simulink model "manning_test_su_nonlinear"  (R2022b)
settings: Solver=VariableStepAuto  StartTime=0.0  StopTime=5*N  RelTol=1e-3
values from neighbouring files (symbols this model uses):
  yd_ds = ss(yd_ds)    [manning_test.m]
  yu_ds = ss(yu_ds)    [manning_test.m]
settings Model: Creator=chuan  LastModifiedBy=chuan

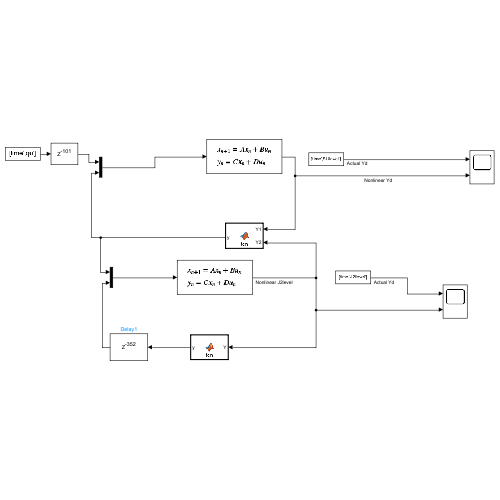
[thumbnail: Simulink's stored preview of the top-level diagram]
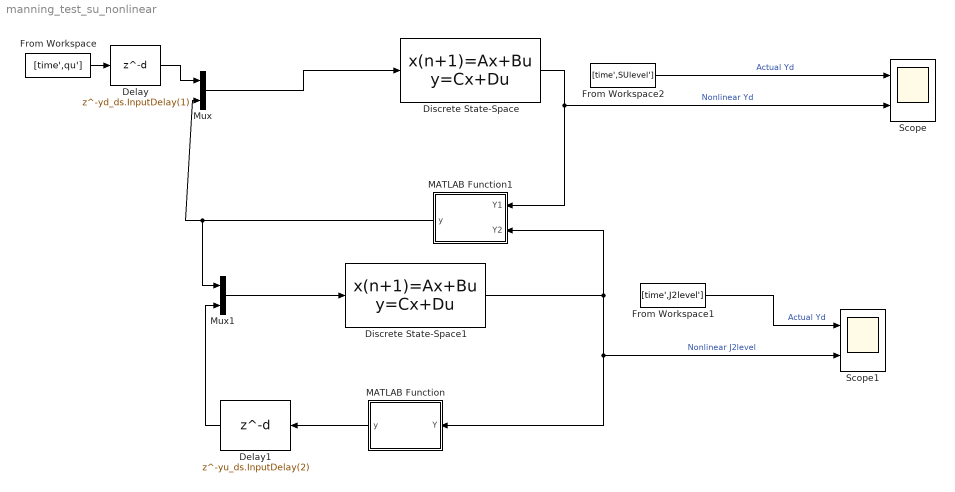
== system manning_test_su_nonlinear ==
  Delay : Delay  DelayLength=yd_ds.InputDelay(1)  InitialCondition=0
  Delay1 : Delay  DelayLength=yu_ds.InputDelay(2)  InitialCondition=0
  Discrete State-Space : DiscreteStateSpace  A=yd_ds.A  B=yd_ds.B  C=yd_ds.C  D=yd_ds.D  SampleTime=yd_ds.Ts
  Discrete State-Space1 : DiscreteStateSpace  A=yu_ds.A  B=yu_ds.B  C=yu_ds.C  D=yu_ds.D  SampleTime=yu_ds.Ts
  From Workspace : FromWorkspace  VariableName=[time',qu']
  From Workspace1 : FromWorkspace  VariableName=[time',J2level']
  From Workspace2 : FromWorkspace  VariableName=[time',SUlevel']
  MATLAB Function : MATLAB Function  TreatAsAtomicUnit=on
  MATLAB Function1 : MATLAB Function  TreatAsAtomicUnit=on
  Mux : Mux  Inputs=2
  Mux1 : Mux  Inputs=2
  Scope : Scope  NumInputPorts=2
  Scope1 : Scope  NumInputPorts=2
  wires:
  Discrete State-Space/1 -> MATLAB Function1/1(Y1), Scope/2  "Nonlinear Yd"
  Mux/1 -> Discrete State-Space/1
  From Workspace2/1 -> Scope/1  "Actual Yd"
  MATLAB Function1/1(y) -> Mux1/1, Mux/2
  Mux1/1 -> Discrete State-Space1/1
  Discrete State-Space1/1 -> MATLAB Function/1(Y), Scope1/2, MATLAB Function1/2(Y2)  "Nonlinear J2level"
  From Workspace1/1 -> Scope1/1  "Actual Yd"
  From Workspace/1 -> Delay/1
  Delay/1 -> Mux/1
  MATLAB Function/1(y) -> Delay1/1
  Delay1/1 -> Mux1/2

== matlab function manning_test_su_nonlinear/MATLAB Function1 ==
  data: Y1 input; y output; Y2 input
function y = fcn(Y1,Y2)
Cd = 0.65;
A0 = 36;
g = 9.81;
Z0 = 5.6;
Yfull = 6;
H_star = Z0 + Yfull;

Y1 = max(Y1,0);
Y2 = max(Y2,0);
H1 = Y1 + Z0;
H2 = Y2 + Z0;

if H1 >= H_star
    if H2 <= Z0 + Yfull/2
        He = H1 - (Z0 + Yfull/2);
    else
        He = H1-H2;
    end

    if He >= 0
        y = Cd*A0*sqrt(2*g*He);
    else
        y = -Cd*A0*sqrt(2*g*-He);
    end
else
    CwL = (Cd*A0*sqrt(g))/(Yfull);
    y = CwL*(H1-Z0)^(1.5);
end

== matlab function manning_test_su_nonlinear/MATLAB Function ==
  data: Y input; y output
function y = fcn(Y)
n = 0.02;
Sb = 0.0008;
B=8;
m = 1.5;

Y = max(Y,0);

y = (1/n)*(B*Y + m*Y.^2)*((B*Y + m*Y.^2)/(B + 2.*Y.*sqrt(1+m^2))).^(2/3) .* sqrt(Sb);
